simulink model "ExoskeletonControlModel"  (R2022b)
settings: Solver=ode3  StartTime=0.0  StopTime=inf  FixedStep=Ts  RelTol=1e-3
PreLoadFcn:
  | Ts_IO204 = 0.001;
  | 
  | if ~exist('Ts', 'var')
  | Ts = 0.001;
  | end
  | if ~exist('FPGA_Frequency', 'var')
  | FPGA_Frequency = 75000000;
  | end
  | 
  | ts_IO612 = 1e-3;
  | 
  | load('TargetReached.mat')
  | load('ActualPos_inc.mat')
model workspace (MAT data in the model file):
  DeltaData : timeseries (value not decoded)
  EC45_deg2incs = 2276
  EC60_deg2inc = 5461
  EC90_deg2incs = 7111
  Enc2rad_18bit = 2.3968e-05
  Enc2rad_19bit = 1.1984e-05
  Enc2rad_20bit = 5.9921e-06
  GiulioModel : robotics.RigidBodyTree (value not decoded)
  Giulio_Spheric_model : robotics.RigidBodyTree (value not decoded)
  Offset1_ticks = 571315
  Offset2_ticks = 590938.9928
  Offset3_ticks = 457912.8279
  Offset4_ticks = 482293.9763
  Offset5_ticks = 598735.9316
  Offset_M1 = 1.12645499896
  Offset_M2 = 4.02728553608
  Offset_M3 = 5.48587511336
  Offset_M4 = 2.03717511516
  Offset_M5 = 4.4996674016
  T1_Nm : object (value not decoded)
  T2_Nm : object (value not decoded)
  TBmodel : robotics.RigidBodyTree (value not decoded)
  Ts = 0.002
  Xg : object (value not decoded)
  Yg : object (value not decoded)
  Zg : object (value not decoded)
  a2 = 0.27
  change_variable = 0
  d1 = [0 0 0 0 0 0 0 0 0 0 0 0 ... (30001 elements, 30001x1)]
  d1_1 = 0.21074
  d2 = [0 0 0 0 0 0 0 0 0 0 0 0 ... (30001 elements, 30001x1)]
  d2_1 = 0.04864
  d3 = [0 0 0 0 0 0 0 0 0 0 0 0 ... (30001 elements, 30001x1)]
  d4 = [0 0 0 0 0 0 0 0 0 0 0 0 ... (30001 elements, 30001x1)]
  d5 = [0 0 0 0 0 0 0 0 0 0 0 0 ... (30001 elements, 30001x1)]
  d6 = [0 0 0 0 0 0 0 0 0 0 0 0 ... (30001 elements, 30001x1)]
  ee_x = -0.2852
  ee_y = -0.3683
  ee_z = -0.0386
  enc2rad_EC45 = 7.6699e-06
  enc2rad_EC90 = 2.3969e-05
  k1_Nm_ticks = 0.00923
  k2_Nm_ticks = 0.0257
  k3_Nm_ticks = 0.00692
  k4_Nm_ticks = 0.00729
  k5_Nm_ticks = 0.00641
  lower_lim_m1 = -330000
  lower_lim_m2 = -235302
  lower_lim_m3 = -132865
  lower_lim_m4 = -152732
  lower_lim_m5 = -138363
  lower_lim_m6 = -200325
  m1 = 2.441408578
  m2 = 3.750007
  m3 = 1.56250298
  m4 = 1.56250298
  m5 = 1.56250298
  m6 = 1.56250298
  n_oversampling = 8
  offset_sea_1 = 0.5547
  offset_sea_2 = 2.8595
  offset_sea_3 = 3.5058
  offset_sea_4 = 2.8586
  offset_sea_5 = 2.8736
  params : AKSIM (value not decoded)
  pos_th_neg = -180000
  pos_th_pos = 180000
  q1 = -1819347
  q2 = -196752
  q3 = -596465
  q4 = -556807
  q5 = -573932
  q6 = -489063
  sine = [0 0.187999937334 0.751998997352 1.69199492401 3.0079839574 4.6999608335 6.76791878442 9.21184953835 12.0317433196 15.2275888485 18.7993733417 22.7470825122 ... (12501 elements, 12501x1)]
  start : object (value not decoded)
  switch_admittance = 1
  t1 : object (value not decoded)
  t2 : object (value not decoded)
  torsionalStiffnes_M1 = 384.88
  torsionalStiffnes_M2 = 1500
  torsionalStiffnes_M3 = 901.97
  torsionalStiffnes_M4 = 950.86
  torsionalStiffnes_M5 = 930
  torsionalStiffnes_M6 = 914
  upper_lim_m1 = 340000
  upper_lim_m2 = 95467
  upper_lim_m3 = 164951
  upper_lim_m4 = 210607
  upper_lim_m5 = 252595
  upper_lim_m6 = 96694
  vel_th_neg = -100
  vel_th_pos = 100
  x = 0
undefined symbols (not defined in the file): C, DiscIntNeverNeededParam
libraries: canmsglib x285, speedgoatlib_IO614 x245, simulink x26, slrealtimeloglib x9, simulink_extras x6, robotmaniplib x6
(part 5 of 13)

== system ExoskeletonControlModel/DataProcessing/CST_trasparency/SendTorqueCommand ==
  note: SEND TORQUE COMMANDS TO EPOS
  In1 : Inport
  TAU_M6 : Inport  Port=2
  TAU_M5 : Inport  Port=3
  TAU_M4 : Inport  Port=4
  TAU_M3 : Inport  Port=5
  In6 : Inport  Port=6
  Gain : Gain  Gain=1/100
  Rate Transition4 : RateTransition  Deterministic=off  OutPortSampleTime=Ts
  Subsystem : Subsystem
  Subsystem1 : Subsystem
  Subsystem2 : Subsystem
  Subsystem3 : Subsystem
  Subsystem4 : Subsystem
  Thousands of nominal torque EC1 : Gain  Gain=-2341
  wires:
  TAU_M6/1 -> Subsystem/1(TAU_M6)
  TAU_M4/1 -> Subsystem1/1(TAU_M4)  "target_torque_m4"
  TAU_M5/1 -> Subsystem2/1(TAU_M5)  "target_torque_m5"
  TAU_M3/1 -> Subsystem3/1(TAU_M3)  "target_torque_m3"
  In1/1 -> Subsystem4/Enable, Subsystem3/Enable, Subsystem1/Enable, Subsystem2/Enable, Subsystem/Enable
  In6/1 -> Thousands of nominal torque EC1/1  "target_torque_m1"
  Thousands of nominal torque EC1/1 -> Gain/1  "Reference Drive Current | Volt"
  Gain/1 -> Rate Transition4/1  "Reference Drive Current | Volt"
  Rate Transition4/1 -> Subsystem4/1(target_torque_m1)

== system ExoskeletonControlModel/DataProcessing/Coupling/receive_PDO3_m2 ==
  target_pos : Inport
  CAN Write : speedgoatlib_IO614/CAN/CAN Write  id=1  sampleTime=-1  portSelection=3  messageType=CAN  enaStatusPort=off  protl=IO614  ptIdx=2  isFDMod=0
  set_position : canmsglib/CAN Pack  MsgList=(none)  MsgName=CAN Msg  MsgIDType=Standard (11-bit identifier)  MsgIdentifier=hex2dec('402')  MsgLength=4  Remote=off  ApplyMinMax=off  BusOutput=off  SignalInfo={ 'target position', '0', '32', 'LE', 'signed', 'Standard', '0', '1', '0', '-Inf', 'Inf' }
      settings: DataFormat=manually specified signals
  wires:
  target_pos/1 -> set_position/1
  set_position/1 -> CAN Write/1

== system ExoskeletonControlModel/DataProcessing/GravityCompensationTorqueComputation/Joints_degrees ==
  PDO_M1_M2_M3_M4_M5_M6 : Inport
  Bus Selector : BusSelector  OutputSignals=PDO_M1.pos_actual_1,PDO_M2.pos_actual_2,PDO_M3.pos_actual_3,PDO_M4.pos_actual_4,PDO_M5.pos_actual_5,PDO_M6.pos_actual_6
  Constant : Constant  Value=-17086
  Constant1 : Constant  Value=13637
  Constant2 : Constant  Value=50153
  Constant3 : Constant  Value=-22699
  Constant4 : Constant  Value=-9784
  Constant5 : Constant  Value=-165590
  Gain1 : Gain  Gain=1/EC45_deg2incs
  Gain12 : Gain  Gain=-1/EC60_deg2inc
  Gain2 : Gain  Gain=-1/EC45_deg2incs
  Gain3 : Gain  Gain=1/EC45_deg2incs
  Gain4 : Gain  Gain=1/EC45_deg2incs
  Gain5 : Gain  Gain=-1/EC90_deg2incs
  JOINTS_DEGREE : slrealtimeloglib/File Log  decimation=1  inputProcessing=Elements as channels (sample based)
  Mux : Mux  Inputs=6
  Sum{,1..5} (6 alike) : Sum  Inputs=|+-
  wires:
  Gain2/1 -> Mux/4  "j4_deg"
  Gain12/1 -> Mux/2  "j2_deg"
  PDO_M1_M2_M3_M4_M5_M6/1 -> Bus Selector/1
  Gain3/1 -> Mux/5  "j5_deg"
  Gain5/1 -> Mux/1  "j1_deg"
  Gain4/1 -> Mux/6  "j6_deg"
  Gain1/1 -> Mux/3  "j3_deg"
  Mux/1 -> JOINTS_DEGREE/1
  Bus Selector/1 -> Sum/1  "<pos_actual_1>"
  Sum/1 -> Gain5/1
  Constant/1 -> Sum/2
  Sum2/1 -> Gain1/1
  Sum1/1 -> Gain12/1
  Sum3/1 -> Gain2/1
  Sum4/1 -> Gain3/1
  Sum5/1 -> Gain4/1
  Bus Selector/2 -> Sum1/1  "<pos_actual_2>"
  Bus Selector/3 -> Sum2/1  "<pos_actual_3>"
  Bus Selector/4 -> Sum3/1  "<pos_actual_4>"
  Bus Selector/5 -> Sum4/1  "<pos_actual_5>"
  Bus Selector/6 -> Sum5/1  "<pos_actual_6>"
  Constant1/1 -> Sum1/2
  Constant2/1 -> Sum2/2
  Constant3/1 -> Sum3/2
  Constant4/1 -> Sum4/2
  Constant5/1 -> Sum5/2

== system ExoskeletonControlModel/DataProcessing/Homing_State_Machine/Homing_m1/FAULT.Fault_reset ==
  note: MOTOR 1 - CONTROLWORD
  Action Port : ActionPort
      settings: CopyFcn=Stateflow.SLINSF.SimulinkMan.removeBlockPreDeleteFcn  PreDeleteFcn=Stateflow.SLINSF.SimulinkMan.unsafePredeleteFcn
  controlword_m1 : Constant  Value=128
  receive_PDO1_m1 : Subsystem
  wires:
  controlword_m1/1 -> receive_PDO1_m1/1(controlword)

== system ExoskeletonControlModel/DataProcessing/Homing_State_Machine/Homing_m1/FAULT.ST4_shutdown ==
  note: MOTOR 1 - CONTROLWORD
  Action Port : ActionPort
      settings: CopyFcn=Stateflow.SLINSF.SimulinkMan.removeBlockPreDeleteFcn  PreDeleteFcn=Stateflow.SLINSF.SimulinkMan.unsafePredeleteFcn
  controlword_m1 : Constant  Value=6
  receive_PDO1_m1 : Subsystem
  wires:
  controlword_m1/1 -> receive_PDO1_m1/1(controlword)

== system ExoskeletonControlModel/DataProcessing/Homing_State_Machine/Homing_m1/HOMING.ST10_set_PPM ==
  note: MOTOR 1 - MODE & INTERPOLATION TIME PERIOD
  Action Port : ActionPort
      settings: CopyFcn=Stateflow.SLINSF.SimulinkMan.removeBlockPreDeleteFcn  PreDeleteFcn=Stateflow.SLINSF.SimulinkMan.unsafePredeleteFcn
  Bus Creator3 : BusCreator  Inputs=2
  interpolation_period_m1 : Constant  Value=10
  mode_m1 : Constant
  receive_PDO2_m1 : Subsystem
  wires:
  Bus Creator3/1 -> receive_PDO2_m1/1(mode)
  mode_m1/1 -> Bus Creator3/1  "mode_m1"
  interpolation_period_m1/1 -> Bus Creator3/2  "interpolation_period_m1"

== system ExoskeletonControlModel/DataProcessing/Homing_State_Machine/Homing_m1/HOMING.ST11_shutdown1 ==
  note: MOTOR 1 - CONTROLWORD
  Action Port : ActionPort
      settings: CopyFcn=Stateflow.SLINSF.SimulinkMan.removeBlockPreDeleteFcn  PreDeleteFcn=Stateflow.SLINSF.SimulinkMan.unsafePredeleteFcn
  controlword_m1 : Constant  Value=6
  receive_PDO1_m1 : Subsystem
  wires:
  controlword_m1/1 -> receive_PDO1_m1/1(controlword)

== system ExoskeletonControlModel/DataProcessing/Homing_State_Machine/Homing_m1/HOMING.ST12_Switch_on_and_Enable_Operation ==
  note: MOTOR 1 - CONTROLWORD
  Action Port : ActionPort
      settings: CopyFcn=Stateflow.SLINSF.SimulinkMan.removeBlockPreDeleteFcn  PreDeleteFcn=Stateflow.SLINSF.SimulinkMan.unsafePredeleteFcn
  controlword_m1 : Constant  Value=15
  receive_PDO1_m1 : Subsystem
  wires:
  controlword_m1/1 -> receive_PDO1_m1/1(controlword)

== system ExoskeletonControlModel/DataProcessing/Homing_State_Machine/Homing_m1/HOMING.ST13_send_target_pos ==
  note: MOTOR 1 - TARGET POSITION
  Action Port : ActionPort
      settings: CopyFcn=Stateflow.SLINSF.SimulinkMan.removeBlockPreDeleteFcn  PreDeleteFcn=Stateflow.SLINSF.SimulinkMan.unsafePredeleteFcn
  receive_PDO3_m1 : Subsystem
  target_position_m1 : Constant  Value=0
  wires:
  target_position_m1/1 -> receive_PDO3_m1/1(target_pos)

== system ExoskeletonControlModel/DataProcessing/Homing_State_Machine/Homing_m1/HOMING.ST14_Abs_ref_start_immediatly ==
  note: MOTOR 1 - CONTROLWORD
  Action Port : ActionPort
      settings: CopyFcn=Stateflow.SLINSF.SimulinkMan.removeBlockPreDeleteFcn  PreDeleteFcn=Stateflow.SLINSF.SimulinkMan.unsafePredeleteFcn
  controlword_m1 : Constant  Value=63
  receive_PDO1_m1 : Subsystem
  wires:
  controlword_m1/1 -> receive_PDO1_m1/1(controlword)

== system ExoskeletonControlModel/DataProcessing/Homing_State_Machine/Homing_m1/HOMING.ST15_set_home_mode ==
  note: MOTOR 1 - MODE & INTERPOLATION TIME PERIOD
  Action Port : ActionPort
      settings: CopyFcn=Stateflow.SLINSF.SimulinkMan.removeBlockPreDeleteFcn  PreDeleteFcn=Stateflow.SLINSF.SimulinkMan.unsafePredeleteFcn
  Bus Creator3 : BusCreator  Inputs=2
  interpolation_period_m1 : Constant  Value=10
  mode_m1 : Constant  Value=6
  receive_PDO2_m1 : Subsystem
  wires:
  Bus Creator3/1 -> receive_PDO2_m1/1(mode)
  mode_m1/1 -> Bus Creator3/1  "mode_m1"
  interpolation_period_m1/1 -> Bus Creator3/2  "interpolation_period_m1"

== system ExoskeletonControlModel/DataProcessing/Homing_State_Machine/Homing_m1/HOMING.ST1_Enter_Pre_Operational ==
  Action Port : ActionPort
      settings: CopyFcn=Stateflow.SLINSF.SimulinkMan.removeBlockPreDeleteFcn  PreDeleteFcn=Stateflow.SLINSF.SimulinkMan.unsafePredeleteFcn
  CS : Constant  Value=128
  set_NMT_state : Subsystem
  wires:
  CS/1 -> set_NMT_state/1(Input)

== system ExoskeletonControlModel/DataProcessing/Homing_State_Machine/Homing_m1/HOMING.ST2_operational ==
  Action Port : ActionPort
      settings: CopyFcn=Stateflow.SLINSF.SimulinkMan.removeBlockPreDeleteFcn  PreDeleteFcn=Stateflow.SLINSF.SimulinkMan.unsafePredeleteFcn
  CS : Constant
  set_NMT_state : Subsystem
  wires:
  CS/1 -> set_NMT_state/1(Input)

== system ExoskeletonControlModel/DataProcessing/Homing_State_Machine/Homing_m1/HOMING.ST3_set_home_mode ==
  note: MOTOR 1 - MODE & INTERPOLATION TIME PERIOD
  Action Port : ActionPort
      settings: CopyFcn=Stateflow.SLINSF.SimulinkMan.removeBlockPreDeleteFcn  PreDeleteFcn=Stateflow.SLINSF.SimulinkMan.unsafePredeleteFcn
  Bus Creator3 : BusCreator  Inputs=2
  interpolation_period_m1 : Constant  Value=10
  mode_m1 : Constant  Value=6
  receive_PDO2_m1 : Subsystem
  wires:
  Bus Creator3/1 -> receive_PDO2_m1/1(mode)
  mode_m1/1 -> Bus Creator3/1  "mode_m1"
  interpolation_period_m1/1 -> Bus Creator3/2  "interpolation_period_m1"

== system ExoskeletonControlModel/DataProcessing/Homing_State_Machine/Homing_m1/HOMING.ST4_shutdown ==
  note: MOTOR 1 - CONTROLWORD
  Action Port : ActionPort
      settings: CopyFcn=Stateflow.SLINSF.SimulinkMan.removeBlockPreDeleteFcn  PreDeleteFcn=Stateflow.SLINSF.SimulinkMan.unsafePredeleteFcn
  controlword_m1 : Constant  Value=6
  receive_PDO1_m1 : Subsystem
  wires:
  controlword_m1/1 -> receive_PDO1_m1/1(controlword)

== system ExoskeletonControlModel/DataProcessing/Homing_State_Machine/Homing_m1/HOMING.ST5_Switch_on_and_Enable_Operation ==
  note: MOTOR 1 - CONTROLWORD
  Action Port : ActionPort
      settings: CopyFcn=Stateflow.SLINSF.SimulinkMan.removeBlockPreDeleteFcn  PreDeleteFcn=Stateflow.SLINSF.SimulinkMan.unsafePredeleteFcn
  controlword_m1 : Constant  Value=15
  receive_PDO1_m1 : Subsystem
  wires:
  controlword_m1/1 -> receive_PDO1_m1/1(controlword)

== system ExoskeletonControlModel/DataProcessing/Homing_State_Machine/Homing_m1/HOMING.ST6_set_home_position ==
  pos_ticks : Inport
  Action Port : ActionPort
      settings: CopyFcn=Stateflow.SLINSF.SimulinkMan.removeBlockPreDeleteFcn  PreDeleteFcn=Stateflow.SLINSF.SimulinkMan.unsafePredeleteFcn
  CAN Write : speedgoatlib_IO614/CAN/CAN Write  id=1  sampleTime=-1  portSelection=3  messageType=CAN  enaStatusPort=off  protl=IO614  ptIdx=2  isFDMod=0
  CS : Constant  Value=hex2dec('22')
  Index : Constant  Value=hex2dec('30B0')
  SubIndex : Constant  Value=hex2dec('00')
  rxSDO : canmsglib/CAN Pack  MsgList=(none)  MsgName=CAN Msg  MsgIDType=Standard (11-bit identifier)  MsgIdentifier=1537  MsgLength=8  Remote=off  ApplyMinMax=off  BusOutput=off  SignalInfo={ 'CS', '0', '8', 'LE', 'unsigned', 'Standard', '0', '1', '0', '-Inf', 'Inf'; 'Index', '8', '16', 'LE', 'unsigned', 'Standard', '0', '1', '0', '-Inf', 'Inf'; 'SubIndex', '24', '8', 'LE', 'unsigned', 'Standard', '0', '1', '0', '-Inf', 'Inf'; 'ParamData', '32', '32', 'LE', 'signed', 'Standard', '0', '1', '0', '-Inf', 'Inf' }
      settings: DataFormat=manually specified signals
  wires:
  SubIndex/1 -> rxSDO/3
  CS/1 -> rxSDO/1
  Index/1 -> rxSDO/2
  rxSDO/1 -> CAN Write/1
  pos_ticks/1 -> rxSDO/4

== system ExoskeletonControlModel/DataProcessing/Homing_State_Machine/Homing_m1/HOMING.ST7_set_home_method ==
  Action Port : ActionPort
      settings: CopyFcn=Stateflow.SLINSF.SimulinkMan.removeBlockPreDeleteFcn  PreDeleteFcn=Stateflow.SLINSF.SimulinkMan.unsafePredeleteFcn
  CAN Write : speedgoatlib_IO614/CAN/CAN Write  id=1  sampleTime=-1  portSelection=3  messageType=CAN  enaStatusPort=off  protl=IO614  ptIdx=2  isFDMod=0
  CS : Constant  Value=hex2dec('22')
  Index : Constant  Value=hex2dec('6098')
  ParamData : Constant  Value=37
  SubIndex : Constant  Value=hex2dec('00')
  rxSDO : canmsglib/CAN Pack  MsgList=(none)  MsgName=CAN Msg  MsgIDType=Standard (11-bit identifier)  MsgIdentifier=1537  MsgLength=8  Remote=off  ApplyMinMax=off  BusOutput=off  SignalInfo={ 'CS', '0', '8', 'LE', 'unsigned', 'Standard', '0', '1', '0', '-Inf', 'Inf'; 'Index', '8', '16', 'LE', 'unsigned', 'Standard', '0', '1', '0', '-Inf', 'Inf'; 'SubIndex', '24', '8', 'LE', 'unsigned', 'Standard', '0', '1', '0', '-Inf', 'Inf'; 'ParamData', '32', '32', 'LE', 'unsigned', 'Standard', '0', '1', '0', '-Inf', 'Inf' }
      settings: DataFormat=manually specified signals
  wires:
  ParamData/1 -> rxSDO/4
  Index/1 -> rxSDO/2
  CS/1 -> rxSDO/1
  SubIndex/1 -> rxSDO/3
  rxSDO/1 -> CAN Write/1

== system ExoskeletonControlModel/DataProcessing/Homing_State_Machine/Homing_m1/HOMING.ST8_start_homing ==
  note: MOTOR 1 - CONTROLWORD
  Action Port : ActionPort
      settings: CopyFcn=Stateflow.SLINSF.SimulinkMan.removeBlockPreDeleteFcn  PreDeleteFcn=Stateflow.SLINSF.SimulinkMan.unsafePredeleteFcn
  controlword_m1 : Constant  Value=31
  receive_PDO1_m1 : Subsystem
  wires:
  controlword_m1/1 -> receive_PDO1_m1/1(controlword)

== system ExoskeletonControlModel/DataProcessing/Homing_State_Machine/Homing_m1/HOMING.ST9_stop_homing ==
  note: MOTOR 1 - CONTROLWORD
  Action Port : ActionPort
      settings: CopyFcn=Stateflow.SLINSF.SimulinkMan.removeBlockPreDeleteFcn  PreDeleteFcn=Stateflow.SLINSF.SimulinkMan.unsafePredeleteFcn
  controlword_m1 : Constant  Value=15
  receive_PDO1_m1 : Subsystem
  wires:
  controlword_m1/1 -> receive_PDO1_m1/1(controlword)

== system ExoskeletonControlModel/DataProcessing/Homing_State_Machine/Homing_m1/HOMING.ST_SET_ACC_LIMITS ==
  Action Port : ActionPort
      settings: CopyFcn=Stateflow.SLINSF.SimulinkMan.removeBlockPreDeleteFcn  PreDeleteFcn=Stateflow.SLINSF.SimulinkMan.unsafePredeleteFcn
  CAN Write : speedgoatlib_IO614/CAN/CAN Write  id=1  sampleTime=-1  portSelection=3  messageType=CAN  enaStatusPort=off  protl=IO614  ptIdx=2  isFDMod=0
  CS : Constant  Value=hex2dec('22')
  Index : Constant  Value=hex2dec('6083')
  ParamData : Constant  Value=100
  SubIndex : Constant  Value=hex2dec('00')
  rxSDO : canmsglib/CAN Pack  MsgList=(none)  MsgName=CAN Msg  MsgIDType=Standard (11-bit identifier)  MsgIdentifier=1537  MsgLength=8  Remote=off  ApplyMinMax=off  BusOutput=off  SignalInfo={ 'CS', '0', '8', 'LE', 'unsigned', 'Standard', '0', '1', '0', '-Inf', 'Inf'; 'Index', '8', '16', 'LE', 'unsigned', 'Standard', '0', '1', '0', '-Inf', 'Inf'; 'SubIndex', '24', '8', 'LE', 'unsigned', 'Standard', '0', '1', '0', '-Inf', 'Inf'; 'ParamData', '32', '32', 'LE', 'unsigned', 'Standard', '0', '1', '0', '-Inf', 'Inf' }
      settings: DataFormat=manually specified signals
  wires:
  ParamData/1 -> rxSDO/4
  Index/1 -> rxSDO/2
  CS/1 -> rxSDO/1
  SubIndex/1 -> rxSDO/3
  rxSDO/1 -> CAN Write/1

== system ExoskeletonControlModel/DataProcessing/Homing_State_Machine/Homing_m1/HOMING.ST_SET_POS_HIGH_LIMITS ==
  Action Port : ActionPort
      settings: CopyFcn=Stateflow.SLINSF.SimulinkMan.removeBlockPreDeleteFcn  PreDeleteFcn=Stateflow.SLINSF.SimulinkMan.unsafePredeleteFcn
  CAN Write : speedgoatlib_IO614/CAN/CAN Write  id=1  sampleTime=-1  portSelection=3  messageType=CAN  enaStatusPort=off  protl=IO614  ptIdx=2  isFDMod=0
  CS : Constant  Value=hex2dec('22')
  Index : Constant  Value=hex2dec('607D')
  ParamData : Constant  Value=upper_lim_m1
  SubIndex : Constant  Value=hex2dec('02')
  rxSDO : canmsglib/CAN Pack  MsgList=(none)  MsgName=CAN Msg  MsgIDType=Standard (11-bit identifier)  MsgIdentifier=1537  MsgLength=8  Remote=off  ApplyMinMax=off  BusOutput=off  SignalInfo={ 'CS', '0', '8', 'LE', 'unsigned', 'Standard', '0', '1', '0', '-Inf', 'Inf'; 'Index', '8', '16', 'LE', 'unsigned', 'Standard', '0', '1', '0', '-Inf', 'Inf'; 'SubIndex', '24', '8', 'LE', 'unsigned', 'Standard', '0', '1', '0', '-Inf', 'Inf'; 'ParamData', '32', '32', 'LE', 'signed', 'Standard', '0', '1', '0', '-Inf', 'Inf' }
      settings: DataFormat=manually specified signals
  wires:
  ParamData/1 -> rxSDO/4
  Index/1 -> rxSDO/2
  CS/1 -> rxSDO/1
  SubIndex/1 -> rxSDO/3
  rxSDO/1 -> CAN Write/1

== system ExoskeletonControlModel/DataProcessing/Homing_State_Machine/Homing_m1/HOMING.ST_SET_POS_LOW_LIMITS ==
  Action Port : ActionPort
      settings: CopyFcn=Stateflow.SLINSF.SimulinkMan.removeBlockPreDeleteFcn  PreDeleteFcn=Stateflow.SLINSF.SimulinkMan.unsafePredeleteFcn
  CAN Write : speedgoatlib_IO614/CAN/CAN Write  id=1  sampleTime=-1  portSelection=3  messageType=CAN  enaStatusPort=off  protl=IO614  ptIdx=2  isFDMod=0
  CS : Constant  Value=hex2dec('22')
  Index : Constant  Value=hex2dec('607D')
  ParamData : Constant  Value=lower_lim_m1
  SubIndex : Constant  Value=hex2dec('01')
  rxSDO : canmsglib/CAN Pack  MsgList=(none)  MsgName=CAN Msg  MsgIDType=Standard (11-bit identifier)  MsgIdentifier=1537  MsgLength=8  Remote=off  ApplyMinMax=off  BusOutput=off  SignalInfo={ 'CS', '0', '8', 'LE', 'unsigned', 'Standard', '0', '1', '0', '-Inf', 'Inf'; 'Index', '8', '16', 'LE', 'unsigned', 'Standard', '0', '1', '0', '-Inf', 'Inf'; 'SubIndex', '24', '8', 'LE', 'unsigned', 'Standard', '0', '1', '0', '-Inf', 'Inf'; 'ParamData', '32', '32', 'LE', 'signed', 'Standard', '0', '1', '0', '-Inf', 'Inf' }
      settings: DataFormat=manually specified signals
  wires:
  ParamData/1 -> rxSDO/4
  Index/1 -> rxSDO/2
  CS/1 -> rxSDO/1
  SubIndex/1 -> rxSDO/3
  rxSDO/1 -> CAN Write/1

== system ExoskeletonControlModel/DataProcessing/Homing_State_Machine/Homing_m1/HOMING.ST_SET_SPEED_LIMITS ==
  Action Port : ActionPort
      settings: CopyFcn=Stateflow.SLINSF.SimulinkMan.removeBlockPreDeleteFcn  PreDeleteFcn=Stateflow.SLINSF.SimulinkMan.unsafePredeleteFcn
  CAN Write : speedgoatlib_IO614/CAN/CAN Write  id=1  sampleTime=-1  portSelection=3  messageType=CAN  enaStatusPort=off  protl=IO614  ptIdx=2  isFDMod=0
  CS : Constant  Value=hex2dec('22')
  Index : Constant  Value=hex2dec('6081')
  ParamData : Constant  Value=100
  SubIndex : Constant  Value=hex2dec('00')
  rxSDO : canmsglib/CAN Pack  MsgList=(none)  MsgName=CAN Msg  MsgIDType=Standard (11-bit identifier)  MsgIdentifier=1537  MsgLength=8  Remote=off  ApplyMinMax=off  BusOutput=off  SignalInfo={ 'CS', '0', '8', 'LE', 'unsigned', 'Standard', '0', '1', '0', '-Inf', 'Inf'; 'Index', '8', '16', 'LE', 'unsigned', 'Standard', '0', '1', '0', '-Inf', 'Inf'; 'SubIndex', '24', '8', 'LE', 'unsigned', 'Standard', '0', '1', '0', '-Inf', 'Inf'; 'ParamData', '32', '32', 'LE', 'unsigned', 'Standard', '0', '1', '0', '-Inf', 'Inf' }
      settings: DataFormat=manually specified signals
  wires:
  ParamData/1 -> rxSDO/4
  Index/1 -> rxSDO/2
  CS/1 -> rxSDO/1
  SubIndex/1 -> rxSDO/3
  rxSDO/1 -> CAN Write/1

== system ExoskeletonControlModel/DataProcessing/Homing_State_Machine/Homing_m2/FAULT.Fault_reset ==
  note: MOTOR 1 - CONTROLWORD
  Action Port : ActionPort
      settings: CopyFcn=Stateflow.SLINSF.SimulinkMan.removeBlockPreDeleteFcn  PreDeleteFcn=Stateflow.SLINSF.SimulinkMan.unsafePredeleteFcn
  controlword_m1 : Constant  Value=128
  receive_PDO1_m1 : Subsystem
  wires:
  controlword_m1/1 -> receive_PDO1_m1/1(controlword)

== system ExoskeletonControlModel/DataProcessing/Homing_State_Machine/Homing_m2/FAULT.ST4_shutdown ==
  note: MOTOR 1 - CONTROLWORD
  Action Port : ActionPort
      settings: CopyFcn=Stateflow.SLINSF.SimulinkMan.removeBlockPreDeleteFcn  PreDeleteFcn=Stateflow.SLINSF.SimulinkMan.unsafePredeleteFcn
  controlword_m1 : Constant  Value=6
  receive_PDO1_m1 : Subsystem
  wires:
  controlword_m1/1 -> receive_PDO1_m1/1(controlword)

== system ExoskeletonControlModel/DataProcessing/Homing_State_Machine/Homing_m2/HOMING.ST10_set_PPM ==
  note: MOTOR 1 - MODE & INTERPOLATION TIME PERIOD
  Action Port : ActionPort
      settings: CopyFcn=Stateflow.SLINSF.SimulinkMan.removeBlockPreDeleteFcn  PreDeleteFcn=Stateflow.SLINSF.SimulinkMan.unsafePredeleteFcn
  Bus Creator3 : BusCreator  Inputs=2
  interpolation_period_m1 : Constant  Value=10
  mode_m1 : Constant
  receive_PDO2_m1 : Subsystem
  wires:
  Bus Creator3/1 -> receive_PDO2_m1/1(mode)
  mode_m1/1 -> Bus Creator3/1  "mode_m1"
  interpolation_period_m1/1 -> Bus Creator3/2  "interpolation_period_m1"

== system ExoskeletonControlModel/DataProcessing/Homing_State_Machine/Homing_m2/HOMING.ST11_shutdown1 ==
  note: MOTOR 1 - CONTROLWORD
  Action Port : ActionPort
      settings: CopyFcn=Stateflow.SLINSF.SimulinkMan.removeBlockPreDeleteFcn  PreDeleteFcn=Stateflow.SLINSF.SimulinkMan.unsafePredeleteFcn
  controlword_m1 : Constant  Value=6
  receive_PDO1_m1 : Subsystem
  wires:
  controlword_m1/1 -> receive_PDO1_m1/1(controlword)

== system ExoskeletonControlModel/DataProcessing/Homing_State_Machine/Homing_m2/HOMING.ST12_Switch_on_and_Enable_Operation ==
  note: MOTOR 1 - CONTROLWORD
  Action Port : ActionPort
      settings: CopyFcn=Stateflow.SLINSF.SimulinkMan.removeBlockPreDeleteFcn  PreDeleteFcn=Stateflow.SLINSF.SimulinkMan.unsafePredeleteFcn
  controlword_m1 : Constant  Value=15
  receive_PDO1_m1 : Subsystem
  wires:
  controlword_m1/1 -> receive_PDO1_m1/1(controlword)

== system ExoskeletonControlModel/DataProcessing/Homing_State_Machine/Homing_m2/HOMING.ST13_send_target_pos ==
  note: MOTOR 1 - TARGET POSITION
  Action Port : ActionPort
      settings: CopyFcn=Stateflow.SLINSF.SimulinkMan.removeBlockPreDeleteFcn  PreDeleteFcn=Stateflow.SLINSF.SimulinkMan.unsafePredeleteFcn
  receive_PDO3_m1 : Subsystem
  target_position_m1 : Constant  Value=0
  wires:
  target_position_m1/1 -> receive_PDO3_m1/1(target_pos)

== system ExoskeletonControlModel/DataProcessing/Homing_State_Machine/Homing_m2/HOMING.ST14_Abs_ref_start_immediatly ==
  note: MOTOR 1 - CONTROLWORD
  Action Port : ActionPort
      settings: CopyFcn=Stateflow.SLINSF.SimulinkMan.removeBlockPreDeleteFcn  PreDeleteFcn=Stateflow.SLINSF.SimulinkMan.unsafePredeleteFcn
  controlword_m1 : Constant  Value=63
  receive_PDO1_m1 : Subsystem
  wires:
  controlword_m1/1 -> receive_PDO1_m1/1(controlword)

== system ExoskeletonControlModel/DataProcessing/Homing_State_Machine/Homing_m2/HOMING.ST15_set_home_mode ==
  note: MOTOR 1 - MODE & INTERPOLATION TIME PERIOD
  Action Port : ActionPort
      settings: CopyFcn=Stateflow.SLINSF.SimulinkMan.removeBlockPreDeleteFcn  PreDeleteFcn=Stateflow.SLINSF.SimulinkMan.unsafePredeleteFcn
  Bus Creator3 : BusCreator  Inputs=2
  interpolation_period_m1 : Constant  Value=10
  mode_m1 : Constant  Value=6
  receive_PDO2_m1 : Subsystem
  wires:
  Bus Creator3/1 -> receive_PDO2_m1/1(mode)
  mode_m1/1 -> Bus Creator3/1  "mode_m1"
  interpolation_period_m1/1 -> Bus Creator3/2  "interpolation_period_m1"

== system ExoskeletonControlModel/DataProcessing/Homing_State_Machine/Homing_m2/HOMING.ST3_set_home_mode ==
  note: MOTOR 1 - MODE & INTERPOLATION TIME PERIOD
  Action Port : ActionPort
      settings: CopyFcn=Stateflow.SLINSF.SimulinkMan.removeBlockPreDeleteFcn  PreDeleteFcn=Stateflow.SLINSF.SimulinkMan.unsafePredeleteFcn
  Bus Creator3 : BusCreator  Inputs=2
  interpolation_period_m1 : Constant  Value=10
  mode_m1 : Constant  Value=6
  receive_PDO2_m1 : Subsystem
  wires:
  Bus Creator3/1 -> receive_PDO2_m1/1(mode)
  mode_m1/1 -> Bus Creator3/1  "mode_m1"
  interpolation_period_m1/1 -> Bus Creator3/2  "interpolation_period_m1"

== system ExoskeletonControlModel/DataProcessing/Homing_State_Machine/Homing_m2/HOMING.ST4_shutdown ==
  note: MOTOR 1 - CONTROLWORD
  Action Port : ActionPort
      settings: CopyFcn=Stateflow.SLINSF.SimulinkMan.removeBlockPreDeleteFcn  PreDeleteFcn=Stateflow.SLINSF.SimulinkMan.unsafePredeleteFcn
  controlword_m1 : Constant  Value=6
  receive_PDO1_m1 : Subsystem
  wires:
  controlword_m1/1 -> receive_PDO1_m1/1(controlword)

== system ExoskeletonControlModel/DataProcessing/Homing_State_Machine/Homing_m2/HOMING.ST5_Switch_on_and_Enable_Operation ==
  note: MOTOR 1 - CONTROLWORD
  Action Port : ActionPort
      settings: CopyFcn=Stateflow.SLINSF.SimulinkMan.removeBlockPreDeleteFcn  PreDeleteFcn=Stateflow.SLINSF.SimulinkMan.unsafePredeleteFcn
  controlword_m1 : Constant  Value=15
  receive_PDO1_m1 : Subsystem
  wires:
  controlword_m1/1 -> receive_PDO1_m1/1(controlword)

== system ExoskeletonControlModel/DataProcessing/Homing_State_Machine/Homing_m2/HOMING.ST6_set_home_position ==
  pos_ticks : Inport
  Action Port : ActionPort
      settings: CopyFcn=Stateflow.SLINSF.SimulinkMan.removeBlockPreDeleteFcn  PreDeleteFcn=Stateflow.SLINSF.SimulinkMan.unsafePredeleteFcn
  CAN Write : speedgoatlib_IO614/CAN/CAN Write  id=1  sampleTime=-1  portSelection=3  messageType=CAN  enaStatusPort=off  protl=IO614  ptIdx=2  isFDMod=0
  CS : Constant  Value=hex2dec('22')
  Index : Constant  Value=hex2dec('30B0')
  SubIndex : Constant  Value=hex2dec('00')
  rxSDO : canmsglib/CAN Pack  MsgList=(none)  MsgName=CAN Msg  MsgIDType=Standard (11-bit identifier)  MsgIdentifier=1538  MsgLength=8  Remote=off  ApplyMinMax=off  BusOutput=off  SignalInfo={ 'CS', '0', '8', 'LE', 'unsigned', 'Standard', '0', '1', '0', '-Inf', 'Inf'; 'Index', '8', '16', 'LE', 'unsigned', 'Standard', '0', '1', '0', '-Inf', 'Inf'; 'SubIndex', '24', '8', 'LE', 'unsigned', 'Standard', '0', '1', '0', '-Inf', 'Inf'; 'ParamData', '32', '32', 'LE', 'signed', 'Standard', '0', '1', '0', '-Inf', 'Inf' }
      settings: DataFormat=manually specified signals
  wires:
  SubIndex/1 -> rxSDO/3
  CS/1 -> rxSDO/1
  Index/1 -> rxSDO/2
  rxSDO/1 -> CAN Write/1
  pos_ticks/1 -> rxSDO/4

== system ExoskeletonControlModel/DataProcessing/Homing_State_Machine/Homing_m2/HOMING.ST7_set_home_method ==
  Action Port : ActionPort
      settings: CopyFcn=Stateflow.SLINSF.SimulinkMan.removeBlockPreDeleteFcn  PreDeleteFcn=Stateflow.SLINSF.SimulinkMan.unsafePredeleteFcn
  CAN Write : speedgoatlib_IO614/CAN/CAN Write  id=1  sampleTime=-1  portSelection=3  messageType=CAN  enaStatusPort=off  protl=IO614  ptIdx=2  isFDMod=0
  CS : Constant  Value=hex2dec('22')
  Index : Constant  Value=hex2dec('6098')
  ParamData : Constant  Value=37
  SubIndex : Constant  Value=hex2dec('00')
  rxSDO : canmsglib/CAN Pack  MsgList=(none)  MsgName=CAN Msg  MsgIDType=Standard (11-bit identifier)  MsgIdentifier=1538  MsgLength=8  Remote=off  ApplyMinMax=off  BusOutput=off  SignalInfo={ 'CS', '0', '8', 'LE', 'unsigned', 'Standard', '0', '1', '0', '-Inf', 'Inf'; 'Index', '8', '16', 'LE', 'unsigned', 'Standard', '0', '1', '0', '-Inf', 'Inf'; 'SubIndex', '24', '8', 'LE', 'unsigned', 'Standard', '0', '1', '0', '-Inf', 'Inf'; 'ParamData', '32', '32', 'LE', 'unsigned', 'Standard', '0', '1', '0', '-Inf', 'Inf' }
      settings: DataFormat=manually specified signals
  wires:
  ParamData/1 -> rxSDO/4
  Index/1 -> rxSDO/2
  CS/1 -> rxSDO/1
  SubIndex/1 -> rxSDO/3
  rxSDO/1 -> CAN Write/1

== system ExoskeletonControlModel/DataProcessing/Homing_State_Machine/Homing_m2/HOMING.ST8_start_homing ==
  note: MOTOR 1 - CONTROLWORD
  Action Port : ActionPort
      settings: CopyFcn=Stateflow.SLINSF.SimulinkMan.removeBlockPreDeleteFcn  PreDeleteFcn=Stateflow.SLINSF.SimulinkMan.unsafePredeleteFcn
  controlword_m1 : Constant  Value=31
  receive_PDO1_m1 : Subsystem
  wires:
  controlword_m1/1 -> receive_PDO1_m1/1(controlword)

== system ExoskeletonControlModel/DataProcessing/Homing_State_Machine/Homing_m2/HOMING.ST9_stop_homing ==
  note: MOTOR 1 - CONTROLWORD
  Action Port : ActionPort
      settings: CopyFcn=Stateflow.SLINSF.SimulinkMan.removeBlockPreDeleteFcn  PreDeleteFcn=Stateflow.SLINSF.SimulinkMan.unsafePredeleteFcn
  controlword_m1 : Constant  Value=15
  receive_PDO1_m1 : Subsystem
  wires:
  controlword_m1/1 -> receive_PDO1_m1/1(controlword)

== system ExoskeletonControlModel/DataProcessing/Homing_State_Machine/Homing_m2/HOMING.ST_SET_ACC_LIMITS ==
  Action Port : ActionPort
      settings: CopyFcn=Stateflow.SLINSF.SimulinkMan.removeBlockPreDeleteFcn  PreDeleteFcn=Stateflow.SLINSF.SimulinkMan.unsafePredeleteFcn
  CAN Write : speedgoatlib_IO614/CAN/CAN Write  id=1  sampleTime=-1  portSelection=3  messageType=CAN  enaStatusPort=off  protl=IO614  ptIdx=2  isFDMod=0
  CS : Constant  Value=hex2dec('22')
  Index : Constant  Value=hex2dec('6083')
  ParamData : Constant  Value=100
  SubIndex : Constant  Value=hex2dec('00')
  rxSDO : canmsglib/CAN Pack  MsgList=(none)  MsgName=CAN Msg  MsgIDType=Standard (11-bit identifier)  MsgIdentifier=1538  MsgLength=8  Remote=off  ApplyMinMax=off  BusOutput=off  SignalInfo={ 'CS', '0', '8', 'LE', 'unsigned', 'Standard', '0', '1', '0', '-Inf', 'Inf'; 'Index', '8', '16', 'LE', 'unsigned', 'Standard', '0', '1', '0', '-Inf', 'Inf'; 'SubIndex', '24', '8', 'LE', 'unsigned', 'Standard', '0', '1', '0', '-Inf', 'Inf'; 'ParamData', '32', '32', 'LE', 'unsigned', 'Standard', '0', '1', '0', '-Inf', 'Inf' }
      settings: DataFormat=manually specified signals
  wires:
  ParamData/1 -> rxSDO/4
  Index/1 -> rxSDO/2
  CS/1 -> rxSDO/1
  SubIndex/1 -> rxSDO/3
  rxSDO/1 -> CAN Write/1

== system ExoskeletonControlModel/DataProcessing/Homing_State_Machine/Homing_m2/HOMING.ST_SET_POS_HIGH_LIMITS ==
  Action Port : ActionPort
      settings: CopyFcn=Stateflow.SLINSF.SimulinkMan.removeBlockPreDeleteFcn  PreDeleteFcn=Stateflow.SLINSF.SimulinkMan.unsafePredeleteFcn
  CAN Write : speedgoatlib_IO614/CAN/CAN Write  id=1  sampleTime=-1  portSelection=3  messageType=CAN  enaStatusPort=off  protl=IO614  ptIdx=2  isFDMod=0
  CS : Constant  Value=hex2dec('22')
  Index : Constant  Value=hex2dec('607D')
  ParamData : Constant  Value=upper_lim_m2
  SubIndex : Constant  Value=hex2dec('02')
  rxSDO : canmsglib/CAN Pack  MsgList=(none)  MsgName=CAN Msg  MsgIDType=Standard (11-bit identifier)  MsgIdentifier=1538  MsgLength=8  Remote=off  ApplyMinMax=off  BusOutput=off  SignalInfo={ 'CS', '0', '8', 'LE', 'unsigned', 'Standard', '0', '1', '0', '-Inf', 'Inf'; 'Index', '8', '16', 'LE', 'unsigned', 'Standard', '0', '1', '0', '-Inf', 'Inf'; 'SubIndex', '24', '8', 'LE', 'unsigned', 'Standard', '0', '1', '0', '-Inf', 'Inf'; 'ParamData', '32', '32', 'LE', 'signed', 'Standard', '0', '1', '0', '-Inf', 'Inf' }
      settings: DataFormat=manually specified signals
  wires:
  ParamData/1 -> rxSDO/4
  Index/1 -> rxSDO/2
  CS/1 -> rxSDO/1
  SubIndex/1 -> rxSDO/3
  rxSDO/1 -> CAN Write/1

== system ExoskeletonControlModel/DataProcessing/Homing_State_Machine/Homing_m2/HOMING.ST_SET_POS_LOW_LIMITS ==
  Action Port : ActionPort
      settings: CopyFcn=Stateflow.SLINSF.SimulinkMan.removeBlockPreDeleteFcn  PreDeleteFcn=Stateflow.SLINSF.SimulinkMan.unsafePredeleteFcn
  CAN Write : speedgoatlib_IO614/CAN/CAN Write  id=1  sampleTime=-1  portSelection=3  messageType=CAN  enaStatusPort=off  protl=IO614  ptIdx=2  isFDMod=0
  CS : Constant  Value=hex2dec('22')
  Index : Constant  Value=hex2dec('607D')
  ParamData : Constant  Value=lower_lim_m2
  SubIndex : Constant  Value=hex2dec('01')
  rxSDO : canmsglib/CAN Pack  MsgList=(none)  MsgName=CAN Msg  MsgIDType=Standard (11-bit identifier)  MsgIdentifier=1538  MsgLength=8  Remote=off  ApplyMinMax=off  BusOutput=off  SignalInfo={ 'CS', '0', '8', 'LE', 'unsigned', 'Standard', '0', '1', '0', '-Inf', 'Inf'; 'Index', '8', '16', 'LE', 'unsigned', 'Standard', '0', '1', '0', '-Inf', 'Inf'; 'SubIndex', '24', '8', 'LE', 'unsigned', 'Standard', '0', '1', '0', '-Inf', 'Inf'; 'ParamData', '32', '32', 'LE', 'signed', 'Standard', '0', '1', '0', '-Inf', 'Inf' }
      settings: DataFormat=manually specified signals
  wires:
  ParamData/1 -> rxSDO/4
  Index/1 -> rxSDO/2
  CS/1 -> rxSDO/1
  SubIndex/1 -> rxSDO/3
  rxSDO/1 -> CAN Write/1

== system ExoskeletonControlModel/DataProcessing/Homing_State_Machine/Homing_m2/HOMING.ST_SET_SPEED_LIMITS ==
  Action Port : ActionPort
      settings: CopyFcn=Stateflow.SLINSF.SimulinkMan.removeBlockPreDeleteFcn  PreDeleteFcn=Stateflow.SLINSF.SimulinkMan.unsafePredeleteFcn
  CAN Write : speedgoatlib_IO614/CAN/CAN Write  id=1  sampleTime=-1  portSelection=3  messageType=CAN  enaStatusPort=off  protl=IO614  ptIdx=2  isFDMod=0
  CS : Constant  Value=hex2dec('22')
  Index : Constant  Value=hex2dec('6081')
  ParamData : Constant  Value=100
  SubIndex : Constant  Value=hex2dec('00')
  rxSDO : canmsglib/CAN Pack  MsgList=(none)  MsgName=CAN Msg  MsgIDType=Standard (11-bit identifier)  MsgIdentifier=1538  MsgLength=8  Remote=off  ApplyMinMax=off  BusOutput=off  SignalInfo={ 'CS', '0', '8', 'LE', 'unsigned', 'Standard', '0', '1', '0', '-Inf', 'Inf'; 'Index', '8', '16', 'LE', 'unsigned', 'Standard', '0', '1', '0', '-Inf', 'Inf'; 'SubIndex', '24', '8', 'LE', 'unsigned', 'Standard', '0', '1', '0', '-Inf', 'Inf'; 'ParamData', '32', '32', 'LE', 'unsigned', 'Standard', '0', '1', '0', '-Inf', 'Inf' }
      settings: DataFormat=manually specified signals
  wires:
  ParamData/1 -> rxSDO/4
  Index/1 -> rxSDO/2
  CS/1 -> rxSDO/1
  SubIndex/1 -> rxSDO/3
  rxSDO/1 -> CAN Write/1

== system ExoskeletonControlModel/DataProcessing/Homing_State_Machine/Homing_m3/FAULT.Fault_reset ==
  note: MOTOR 1 - CONTROLWORD
  Action Port : ActionPort
      settings: CopyFcn=Stateflow.SLINSF.SimulinkMan.removeBlockPreDeleteFcn  PreDeleteFcn=Stateflow.SLINSF.SimulinkMan.unsafePredeleteFcn
  controlword_m1 : Constant  Value=128
  receive_PDO1_m1 : Subsystem
  wires:
  controlword_m1/1 -> receive_PDO1_m1/1(controlword)

== system ExoskeletonControlModel/DataProcessing/Homing_State_Machine/Homing_m3/FAULT.ST4_shutdown ==
  note: MOTOR 1 - CONTROLWORD
  Action Port : ActionPort
      settings: CopyFcn=Stateflow.SLINSF.SimulinkMan.removeBlockPreDeleteFcn  PreDeleteFcn=Stateflow.SLINSF.SimulinkMan.unsafePredeleteFcn
  controlword_m1 : Constant  Value=6
  receive_PDO1_m1 : Subsystem
  wires:
  controlword_m1/1 -> receive_PDO1_m1/1(controlword)

== system ExoskeletonControlModel/DataProcessing/Homing_State_Machine/Homing_m3/HOMING.ST10_set_PPM ==
  note: MOTOR 1 - MODE & INTERPOLATION TIME PERIOD
  Action Port : ActionPort
      settings: CopyFcn=Stateflow.SLINSF.SimulinkMan.removeBlockPreDeleteFcn  PreDeleteFcn=Stateflow.SLINSF.SimulinkMan.unsafePredeleteFcn
  Bus Creator3 : BusCreator  Inputs=2
  interpolation_period_m1 : Constant  Value=10
  mode_m1 : Constant
  receive_PDO2_m1 : Subsystem
  wires:
  Bus Creator3/1 -> receive_PDO2_m1/1(mode)
  mode_m1/1 -> Bus Creator3/1  "mode_m1"
  interpolation_period_m1/1 -> Bus Creator3/2  "interpolation_period_m1"

== system ExoskeletonControlModel/DataProcessing/Homing_State_Machine/Homing_m3/HOMING.ST11_shutdown1 ==
  note: MOTOR 1 - CONTROLWORD
  Action Port : ActionPort
      settings: CopyFcn=Stateflow.SLINSF.SimulinkMan.removeBlockPreDeleteFcn  PreDeleteFcn=Stateflow.SLINSF.SimulinkMan.unsafePredeleteFcn
  controlword_m1 : Constant  Value=6
  receive_PDO1_m1 : Subsystem
  wires:
  controlword_m1/1 -> receive_PDO1_m1/1(controlword)

== system ExoskeletonControlModel/DataProcessing/Homing_State_Machine/Homing_m3/HOMING.ST12_Switch_on_and_Enable_Operation ==
  note: MOTOR 1 - CONTROLWORD
  Action Port : ActionPort
      settings: CopyFcn=Stateflow.SLINSF.SimulinkMan.removeBlockPreDeleteFcn  PreDeleteFcn=Stateflow.SLINSF.SimulinkMan.unsafePredeleteFcn
  controlword_m1 : Constant  Value=15
  receive_PDO1_m1 : Subsystem
  wires:
  controlword_m1/1 -> receive_PDO1_m1/1(controlword)

== system ExoskeletonControlModel/DataProcessing/Homing_State_Machine/Homing_m3/HOMING.ST13_send_target_pos ==
  note: MOTOR 1 - TARGET POSITION
  Action Port : ActionPort
      settings: CopyFcn=Stateflow.SLINSF.SimulinkMan.removeBlockPreDeleteFcn  PreDeleteFcn=Stateflow.SLINSF.SimulinkMan.unsafePredeleteFcn
  receive_PDO3_m1 : Subsystem
  target_position_m1 : Constant  Value=0
  wires:
  target_position_m1/1 -> receive_PDO3_m1/1(target_pos)

== system ExoskeletonControlModel/DataProcessing/Homing_State_Machine/Homing_m3/HOMING.ST14_Abs_ref_start_immediatly ==
  note: MOTOR 1 - CONTROLWORD
  Action Port : ActionPort
      settings: CopyFcn=Stateflow.SLINSF.SimulinkMan.removeBlockPreDeleteFcn  PreDeleteFcn=Stateflow.SLINSF.SimulinkMan.unsafePredeleteFcn
  controlword_m1 : Constant  Value=63
  receive_PDO1_m1 : Subsystem
  wires:
  controlword_m1/1 -> receive_PDO1_m1/1(controlword)

== system ExoskeletonControlModel/DataProcessing/Homing_State_Machine/Homing_m3/HOMING.ST15_set_home_mode ==
  note: MOTOR 1 - MODE & INTERPOLATION TIME PERIOD
  Action Port : ActionPort
      settings: CopyFcn=Stateflow.SLINSF.SimulinkMan.removeBlockPreDeleteFcn  PreDeleteFcn=Stateflow.SLINSF.SimulinkMan.unsafePredeleteFcn
  Bus Creator3 : BusCreator  Inputs=2
  interpolation_period_m1 : Constant  Value=10
  mode_m1 : Constant  Value=6
  receive_PDO2_m1 : Subsystem
  wires:
  Bus Creator3/1 -> receive_PDO2_m1/1(mode)
  mode_m1/1 -> Bus Creator3/1  "mode_m1"
  interpolation_period_m1/1 -> Bus Creator3/2  "interpolation_period_m1"

== system ExoskeletonControlModel/DataProcessing/Homing_State_Machine/Homing_m3/HOMING.ST1_Enter_Pre_Operational ==
  Action Port : ActionPort
      settings: CopyFcn=Stateflow.SLINSF.SimulinkMan.removeBlockPreDeleteFcn  PreDeleteFcn=Stateflow.SLINSF.SimulinkMan.unsafePredeleteFcn
  CS : Constant  Value=128
  set_NMT_state : Subsystem
  wires:
  CS/1 -> set_NMT_state/1(Input)

== system ExoskeletonControlModel/DataProcessing/Homing_State_Machine/Homing_m3/HOMING.ST2_operational ==
  Action Port : ActionPort
      settings: CopyFcn=Stateflow.SLINSF.SimulinkMan.removeBlockPreDeleteFcn  PreDeleteFcn=Stateflow.SLINSF.SimulinkMan.unsafePredeleteFcn
  CS : Constant
  set_NMT_state : Subsystem
  wires:
  CS/1 -> set_NMT_state/1(Input)

== system ExoskeletonControlModel/DataProcessing/Homing_State_Machine/Homing_m3/HOMING.ST3_set_home_mode ==
  note: MOTOR 1 - MODE & INTERPOLATION TIME PERIOD
  Action Port : ActionPort
      settings: CopyFcn=Stateflow.SLINSF.SimulinkMan.removeBlockPreDeleteFcn  PreDeleteFcn=Stateflow.SLINSF.SimulinkMan.unsafePredeleteFcn
  Bus Creator3 : BusCreator  Inputs=2
  interpolation_period_m1 : Constant  Value=10
  mode_m1 : Constant  Value=6
  receive_PDO2_m1 : Subsystem
  wires:
  Bus Creator3/1 -> receive_PDO2_m1/1(mode)
  mode_m1/1 -> Bus Creator3/1  "mode_m1"
  interpolation_period_m1/1 -> Bus Creator3/2  "interpolation_period_m1"

== system ExoskeletonControlModel/DataProcessing/Homing_State_Machine/Homing_m3/HOMING.ST4_shutdown ==
  note: MOTOR 1 - CONTROLWORD
  Action Port : ActionPort
      settings: CopyFcn=Stateflow.SLINSF.SimulinkMan.removeBlockPreDeleteFcn  PreDeleteFcn=Stateflow.SLINSF.SimulinkMan.unsafePredeleteFcn
  controlword_m1 : Constant  Value=6
  receive_PDO1_m1 : Subsystem
  wires:
  controlword_m1/1 -> receive_PDO1_m1/1(controlword)

== system ExoskeletonControlModel/DataProcessing/Homing_State_Machine/Homing_m3/HOMING.ST5_Switch_on_and_Enable_Operation ==
  note: MOTOR 1 - CONTROLWORD
  Action Port : ActionPort
      settings: CopyFcn=Stateflow.SLINSF.SimulinkMan.removeBlockPreDeleteFcn  PreDeleteFcn=Stateflow.SLINSF.SimulinkMan.unsafePredeleteFcn
  controlword_m1 : Constant  Value=15
  receive_PDO1_m1 : Subsystem
  wires:
  controlword_m1/1 -> receive_PDO1_m1/1(controlword)

== system ExoskeletonControlModel/DataProcessing/Homing_State_Machine/Homing_m3/HOMING.ST6_set_home_position ==
  pos_ticks : Inport
  Action Port : ActionPort
      settings: CopyFcn=Stateflow.SLINSF.SimulinkMan.removeBlockPreDeleteFcn  PreDeleteFcn=Stateflow.SLINSF.SimulinkMan.unsafePredeleteFcn
  CAN Write : speedgoatlib_IO614/CAN/CAN Write  id=1  sampleTime=-1  portSelection=4  messageType=CAN  enaStatusPort=off  protl=IO614  ptIdx=3  isFDMod=0
  CS : Constant  Value=hex2dec('22')
  Index : Constant  Value=hex2dec('30B0')
  SubIndex : Constant  Value=hex2dec('00')
  rxSDO : canmsglib/CAN Pack  MsgList=(none)  MsgName=CAN Msg  MsgIDType=Standard (11-bit identifier)  MsgIdentifier=1537  MsgLength=8  Remote=off  ApplyMinMax=off  BusOutput=off  SignalInfo={ 'CS', '0', '8', 'LE', 'unsigned', 'Standard', '0', '1', '0', '-Inf', 'Inf'; 'Index', '8', '16', 'LE', 'unsigned', 'Standard', '0', '1', '0', '-Inf', 'Inf'; 'SubIndex', '24', '8', 'LE', 'unsigned', 'Standard', '0', '1', '0', '-Inf', 'Inf'; 'ParamData', '32', '32', 'LE', 'signed', 'Standard', '0', '1', '0', '-Inf', 'Inf' }
      settings: DataFormat=manually specified signals
  wires:
  SubIndex/1 -> rxSDO/3
  CS/1 -> rxSDO/1
  Index/1 -> rxSDO/2
  rxSDO/1 -> CAN Write/1
  pos_ticks/1 -> rxSDO/4

== system ExoskeletonControlModel/DataProcessing/Homing_State_Machine/Homing_m3/HOMING.ST7_set_home_method ==
  Action Port : ActionPort
      settings: CopyFcn=Stateflow.SLINSF.SimulinkMan.removeBlockPreDeleteFcn  PreDeleteFcn=Stateflow.SLINSF.SimulinkMan.unsafePredeleteFcn
  CAN Write : speedgoatlib_IO614/CAN/CAN Write  id=1  sampleTime=-1  portSelection=4  messageType=CAN  enaStatusPort=off  protl=IO614  ptIdx=3  isFDMod=0
  CS : Constant  Value=hex2dec('22')
  Index : Constant  Value=hex2dec('6098')
  ParamData : Constant  Value=37
  SubIndex : Constant  Value=hex2dec('00')
  rxSDO : canmsglib/CAN Pack  MsgList=(none)  MsgName=CAN Msg  MsgIDType=Standard (11-bit identifier)  MsgIdentifier=1537  MsgLength=8  Remote=off  ApplyMinMax=off  BusOutput=off  SignalInfo={ 'CS', '0', '8', 'LE', 'unsigned', 'Standard', '0', '1', '0', '-Inf', 'Inf'; 'Index', '8', '16', 'LE', 'unsigned', 'Standard', '0', '1', '0', '-Inf', 'Inf'; 'SubIndex', '24', '8', 'LE', 'unsigned', 'Standard', '0', '1', '0', '-Inf', 'Inf'; 'ParamData', '32', '32', 'LE', 'unsigned', 'Standard', '0', '1', '0', '-Inf', 'Inf' }
      settings: DataFormat=manually specified signals
  wires:
  ParamData/1 -> rxSDO/4
  Index/1 -> rxSDO/2
  CS/1 -> rxSDO/1
  SubIndex/1 -> rxSDO/3
  rxSDO/1 -> CAN Write/1

== system ExoskeletonControlModel/DataProcessing/Homing_State_Machine/Homing_m3/HOMING.ST8_start_homing ==
  note: MOTOR 1 - CONTROLWORD
  Action Port : ActionPort
      settings: CopyFcn=Stateflow.SLINSF.SimulinkMan.removeBlockPreDeleteFcn  PreDeleteFcn=Stateflow.SLINSF.SimulinkMan.unsafePredeleteFcn
  controlword_m1 : Constant  Value=31
  receive_PDO1_m1 : Subsystem
  wires:
  controlword_m1/1 -> receive_PDO1_m1/1(controlword)

== system ExoskeletonControlModel/DataProcessing/Homing_State_Machine/Homing_m3/HOMING.ST9_stop_homing ==
  note: MOTOR 1 - CONTROLWORD
  Action Port : ActionPort
      settings: CopyFcn=Stateflow.SLINSF.SimulinkMan.removeBlockPreDeleteFcn  PreDeleteFcn=Stateflow.SLINSF.SimulinkMan.unsafePredeleteFcn
  controlword_m1 : Constant  Value=15
  receive_PDO1_m1 : Subsystem
  wires:
  controlword_m1/1 -> receive_PDO1_m1/1(controlword)

== system ExoskeletonControlModel/DataProcessing/Homing_State_Machine/Homing_m3/HOMING.ST_SET_ACC_LIMITS ==
  Action Port : ActionPort
      settings: CopyFcn=Stateflow.SLINSF.SimulinkMan.removeBlockPreDeleteFcn  PreDeleteFcn=Stateflow.SLINSF.SimulinkMan.unsafePredeleteFcn
  CAN Write : speedgoatlib_IO614/CAN/CAN Write  id=1  sampleTime=-1  portSelection=4  messageType=CAN  enaStatusPort=off  protl=IO614  ptIdx=3  isFDMod=0
  CS : Constant  Value=hex2dec('22')
  Index : Constant  Value=hex2dec('6083')
  ParamData : Constant  Value=100
  SubIndex : Constant  Value=hex2dec('00')
  rxSDO : canmsglib/CAN Pack  MsgList=(none)  MsgName=CAN Msg  MsgIDType=Standard (11-bit identifier)  MsgIdentifier=1537  MsgLength=8  Remote=off  ApplyMinMax=off  BusOutput=off  SignalInfo={ 'CS', '0', '8', 'LE', 'unsigned', 'Standard', '0', '1', '0', '-Inf', 'Inf'; 'Index', '8', '16', 'LE', 'unsigned', 'Standard', '0', '1', '0', '-Inf', 'Inf'; 'SubIndex', '24', '8', 'LE', 'unsigned', 'Standard', '0', '1', '0', '-Inf', 'Inf'; 'ParamData', '32', '32', 'LE', 'unsigned', 'Standard', '0', '1', '0', '-Inf', 'Inf' }
      settings: DataFormat=manually specified signals
  wires:
  ParamData/1 -> rxSDO/4
  Index/1 -> rxSDO/2
  CS/1 -> rxSDO/1
  SubIndex/1 -> rxSDO/3
  rxSDO/1 -> CAN Write/1

== system ExoskeletonControlModel/DataProcessing/Homing_State_Machine/Homing_m3/HOMING.ST_SET_POS_HIGH_LIMITS ==
  Action Port : ActionPort
      settings: CopyFcn=Stateflow.SLINSF.SimulinkMan.removeBlockPreDeleteFcn  PreDeleteFcn=Stateflow.SLINSF.SimulinkMan.unsafePredeleteFcn
  CAN Write : speedgoatlib_IO614/CAN/CAN Write  id=1  sampleTime=-1  portSelection=4  messageType=CAN  enaStatusPort=off  protl=IO614  ptIdx=3  isFDMod=0
  CS : Constant  Value=hex2dec('22')
  Index : Constant  Value=hex2dec('607D')
  ParamData : Constant  Value=upper_lim_m3
  SubIndex : Constant  Value=hex2dec('02')
  rxSDO : canmsglib/CAN Pack  MsgList=(none)  MsgName=CAN Msg  MsgIDType=Standard (11-bit identifier)  MsgIdentifier=1537  MsgLength=8  Remote=off  ApplyMinMax=off  BusOutput=off  SignalInfo={ 'CS', '0', '8', 'LE', 'unsigned', 'Standard', '0', '1', '0', '-Inf', 'Inf'; 'Index', '8', '16', 'LE', 'unsigned', 'Standard', '0', '1', '0', '-Inf', 'Inf'; 'SubIndex', '24', '8', 'LE', 'unsigned', 'Standard', '0', '1', '0', '-Inf', 'Inf'; 'ParamData', '32', '32', 'LE', 'signed', 'Standard', '0', '1', '0', '-Inf', 'Inf' }
      settings: DataFormat=manually specified signals
  wires:
  ParamData/1 -> rxSDO/4
  Index/1 -> rxSDO/2
  CS/1 -> rxSDO/1
  SubIndex/1 -> rxSDO/3
  rxSDO/1 -> CAN Write/1

== system ExoskeletonControlModel/DataProcessing/Homing_State_Machine/Homing_m3/HOMING.ST_SET_POS_LOW_LIMITS ==
  Action Port : ActionPort
      settings: CopyFcn=Stateflow.SLINSF.SimulinkMan.removeBlockPreDeleteFcn  PreDeleteFcn=Stateflow.SLINSF.SimulinkMan.unsafePredeleteFcn
  CAN Write : speedgoatlib_IO614/CAN/CAN Write  id=1  sampleTime=-1  portSelection=4  messageType=CAN  enaStatusPort=off  protl=IO614  ptIdx=3  isFDMod=0
  CS : Constant  Value=hex2dec('22')
  Index : Constant  Value=hex2dec('607D')
  ParamData : Constant  Value=lower_lim_m3
  SubIndex : Constant  Value=hex2dec('01')
  rxSDO : canmsglib/CAN Pack  MsgList=(none)  MsgName=CAN Msg  MsgIDType=Standard (11-bit identifier)  MsgIdentifier=1537  MsgLength=8  Remote=off  ApplyMinMax=off  BusOutput=off  SignalInfo={ 'CS', '0', '8', 'LE', 'unsigned', 'Standard', '0', '1', '0', '-Inf', 'Inf'; 'Index', '8', '16', 'LE', 'unsigned', 'Standard', '0', '1', '0', '-Inf', 'Inf'; 'SubIndex', '24', '8', 'LE', 'unsigned', 'Standard', '0', '1', '0', '-Inf', 'Inf'; 'ParamData', '32', '32', 'LE', 'signed', 'Standard', '0', '1', '0', '-Inf', 'Inf' }
      settings: DataFormat=manually specified signals
  wires:
  ParamData/1 -> rxSDO/4
  Index/1 -> rxSDO/2
  CS/1 -> rxSDO/1
  SubIndex/1 -> rxSDO/3
  rxSDO/1 -> CAN Write/1
